simulink model "parte2_ej2_GBHP"  (R2019b)
settings: Solver=VariableStepAuto  StartTime=0.0  StopTime=10.0  RelTol=1e-3
values from neighbouring files (symbols this model uses):
  H = 3.5    [parte2_ej2_GeneradorBusInfinito.m]    (also in parte2_ej2_GeneradorBusInfinitoHP.m; parte2_eje2_HPModel.m = 6.5)
  K1 = 0.7643    [parte2_ej2_GeneradorBusInfinitoHP.m]    (also in parte2_eje2_HPModel.m = ((xq-xpd)/(xe+xpd))*iqo*eb*sin(do)+eqo*eb*cos(do)/(xe+xq))
  K2 = 0.8649    [parte2_ej2_GeneradorBusInfinitoHP.m]    (also in parte2_eje2_HPModel.m = eb*sin(do)/(xe+xpd))
  K3 = 0.3230    (= 0.323)    [parte2_ej2_GeneradorBusInfinitoHP.m]    (also in parte2_eje2_HPModel.m = 0.318181818182)
  K4 = 1.4187    [parte2_ej2_GeneradorBusInfinitoHP.m]    (also in parte2_eje2_HPModel.m = (xd-xpd)*sin(do)*eb/(xpd+xe))
  KD = 10    [parte2_ej2_GeneradorBusInfinito.m]    (also in parte2_ej2_GeneradorBusInfinitoHP.m; parte2_eje2_HPModel.m = 0)
  T3 = 2.365    [parte2_ej2_GeneradorBusInfinitoHP.m]    (also in parte2_eje2_HPModel.m = 1.86865341761)
  w0 = 2*pi*60    (= 376.991118431)    [parte2_ej2_GeneradorBusInfinito.m]    (also in parte2_ej2_GeneradorBusInfinitoHP.m; parte2_eje2_HPModel.m)
settings Model: Creator=cjuar  LastModifiedBy=cjuar

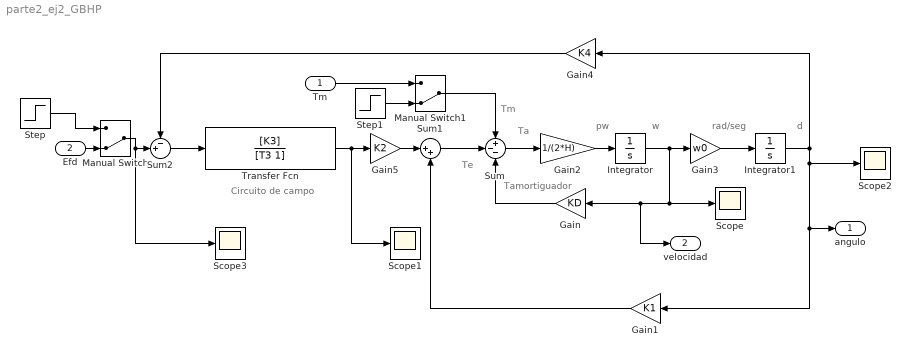
== system parte2_ej2_GBHP ==
  note: Circuito de campo
  note: d
  note: rad/seg
  note: w
  note: pw
  note: Ta
  note: Te
  note: Tamortiguador
  note: Tm
  Tm : Inport
  Efd : Inport  Port=2
  Gain : Gain  Gain=KD
  Gain1 : Gain  Gain=K1
  Gain2 : Gain  Gain=1/(2*H)
  Gain3 : Gain  Gain=w0
  Gain4 : Gain  Gain=K4
  Gain5 : Gain  Gain=K2
  Integrator : Integrator
  Integrator1 : Integrator
  Manual Switch : ManualSwitch  CurrentSetting=0
  Manual Switch1 : ManualSwitch  CurrentSetting=0
  Scope{,1..3} (4 alike) : Scope
  Step : Step  SampleTime=0
  Step1 : Step  SampleTime=0
  Sum : Sum  Inputs=+--
  Sum1 : Sum  Inputs=|++
  Sum2 : Sum  Inputs=-+|
  Transfer Fcn : TransferFcn  Numerator=[K3]  Denominator=[T3 1]
  "angulo " : Outport
  velocidad : Outport  Port=2
  wires:
  Gain/1 -> Sum/3
  Sum/1 -> Gain2/1
  Gain2/1 -> Integrator/1
  Gain3/1 -> Integrator1/1
  Integrator/1 -> Gain3/1, velocidad/1, Gain/1, Scope/1
  Transfer Fcn/1 -> Scope1/1, Gain5/1
  Gain5/1 -> Sum1/1
  Gain1/1 -> Sum1/2
  Gain4/1 -> Sum2/1
  Sum2/1 -> Transfer Fcn/1
  Integrator1/1 -> Scope2/1, "angulo "/1, Gain1/1, Gain4/1
  Sum1/1 -> Sum/2
  Efd/1 -> Manual Switch/2
  Manual Switch/1 -> Scope3/1, Sum2/2
  Step/1 -> Manual Switch/1
  Tm/1 -> Manual Switch1/1
  Manual Switch1/1 -> Sum/1
  Step1/1 -> Manual Switch1/2
